simulink model "Combined_Power_Circuit"  (R2022b)
settings: Solver=VariableStepAuto  StartTime=0.0  StopTime=5  MaxStep=1e-5  RelTol=1e-3
libraries: spsDiodeLib x7, spsACVoltageSourceLib x3, spsCurrentMeasurementLib x3, spsVoltageMeasurementLib x2, spsDCMachineLib x1, spsMeanLib x1, spsMosfetLib x1, spspowerguiLib x1
settings Model: Creator=pc  LastModifiedBy=user
settings SolverCC: ZeroCrossAlgorithm=Adaptive
settings DebuggingCC: IgnoredZcDiagnostic=none  UnconnectedInputMsg=warning  UnconnectedOutputMsg=warning  UnconnectedLineMsg=warning
settings ModelReferenceCC: EnableRefExpFcnMdlSchedulingChecks=on
settings RTWCC: DLArmComputeVersion=19.05

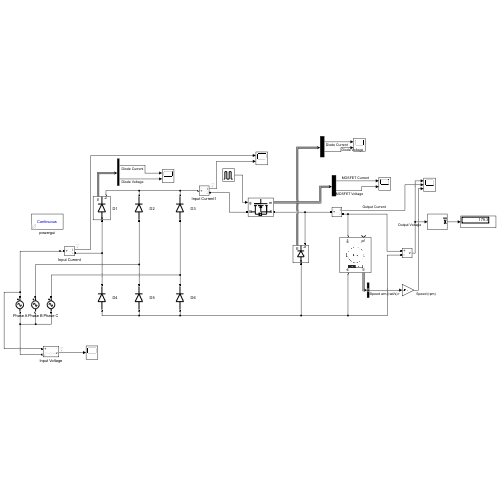
[thumbnail: Simulink's stored preview of the top-level diagram]
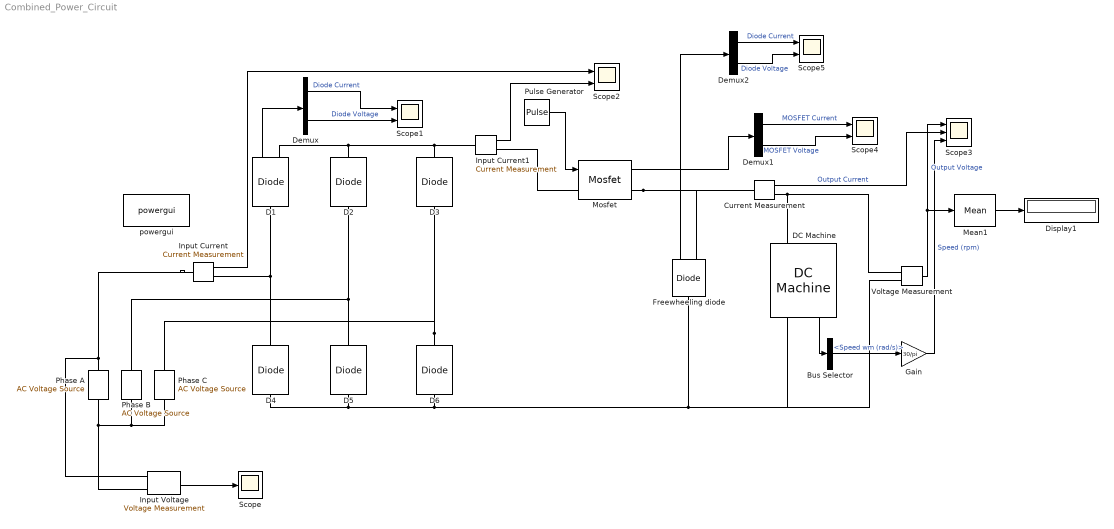
== system Combined_Power_Circuit ==
  " Phase A" : spsACVoltageSourceLib/AC Voltage Source  Amplitude=96.2*sqrt(2)  Phase=0  Frequency=50  SampleTime=0  Measurements=None  BusType=swing  Pref=10e3  Qref=0  Qmin=-inf  Qmax=+inf
  Bus Selector : BusSelector  OutputSignals=Speed wm (rad/s)
  Current Measurement : spsCurrentMeasurementLib/Current Measurement  PhasorSimulation=off  OutputType=Complex  PSBequivalent=0
  D1 : spsDiodeLib/Diode  Ron=0  Lon=0  Vf=0  IC=0  UseSnubber=0  Rs=inf  Cs=0  Measurements=on
  D{2..6} (5 alike) : spsDiodeLib/Diode  Ron=0  Lon=0  Vf=0  IC=0  UseSnubber=0  Rs=inf  Cs=0  Measurements=off
  DC Machine : spsDCMachineLib/DC Machine  PresetModel=No  MechanicalLoad=Torque TL  FieldType=Permanent magnet  ShowDetailedParameters=on  MeasurementBus=off  RLa="[ 0.8  0.0125]"  RLf="[ 210  23]"  Laf=1.8  MachineConstant=Back-emf constant (V/rpm)  Ke=220/1500  Kt=1.8  J=1  Bm=0  Tf=1.59  w0=0  Ifinit=1  TsPowergui=0  TsBlock=-1
  Demux : Demux  Outputs=2
  Demux1 : Demux  Outputs=2
  Demux2 : Demux  Outputs=2
  Display1 : Display
  Freewheeling diode : spsDiodeLib/Diode  Ron=0  Lon=0  Vf=0  IC=0  UseSnubber=off  Rs=inf  Cs=0  Measurements=on
  Gain : Gain  Gain=30/pi
  Input Current : spsCurrentMeasurementLib/Current Measurement  PhasorSimulation=off  OutputType=Complex  PSBequivalent=0
  Input Current1 : spsCurrentMeasurementLib/Current Measurement  PhasorSimulation=off  OutputType=Complex  PSBequivalent=0
  Input Voltage : spsVoltageMeasurementLib/Voltage Measurement  PhasorSimulation=off  OutputType=Complex  PSBequivalent=0
  Mean1 : spsMeanLib/Mean  Freq=60  Vinit=0  Ts=0
  Mosfet : spsMosfetLib/Mosfet  Ron=0.1  Lon=0  Rd=0.01  Vfd=0  IC=0  Rs=1e5  Cs=inf  Measurements=on
  Phase B : spsACVoltageSourceLib/AC Voltage Source  Amplitude=96.2*sqrt(2)  Phase=-120  Frequency=50  SampleTime=0  Measurements=None  BusType=swing  Pref=10e3  Qref=0  Qmin=-inf  Qmax=+inf
  Phase C : spsACVoltageSourceLib/AC Voltage Source  Amplitude=96.2*sqrt(2)  Phase=120  Frequency=50  SampleTime=0  Measurements=None  BusType=swing  Pref=10e3  Qref=0  Qmin=-inf  Qmax=+inf
  Pulse Generator : DiscretePulseGenerator  PulseType=Time based  Period=1/10000  PulseWidth=80
  Scope : Scope
  Scope{1..2,4..5} (4 alike) : Scope  NumInputPorts=2
  Scope3 : Scope  NumInputPorts=3
  Voltage Measurement : spsVoltageMeasurementLib/Voltage Measurement  PhasorSimulation=off  OutputType=Complex  PSBequivalent=0
  powergui : spspowerguiLib/powergui  Priority=1  SimulationMode=Continuous  SampleTime=50e-6  frequency=60  Iterations=50  frequencyindice=50  Pbase=100e6  ErrMax=1e-4  UnitsV=kV  UnitsW=MW  buscounter=0  FunctionMessages=off  echomessages=off  EnableUseOfTLC=off  CurrentSourceSwitches=off  DisableSnubberDevices=off  DisableRonSwitches=off  DisableVfSwitches=off  DisplayEquations=off  AutomaticDiscreteSolvers=off  SolverType=Tustin/Backward Euler (TBE)  Interpol=off  ExternalGateDelay=off  methode=off  Ts=100  x0status=blocks  SPID=on  SwTol=0  HookPort=off  NonlinearTolerance=1e-4  nMaxIteration=100  ContinueOnMaxIteration=off  RestoreLinks=warning  ResistiveCurrentMeasurement=off  Frange=[0:2:500]  Ylog=off  Xlog=on  ShowGrid=off  save=off  variable=ZData  structure=0  ZoomFFT=off  StartTime=0.0  cycles=1  DisplayStyle=1  fundamental=60  FreqAxis=off  MaxFrequency=1000  frequencyindicesteady=1  RmsSteady=1  display=off
  wires:
  Input Voltage/1 -> Scope/1
  D1/1 -> Demux/1
  Demux/1 -> Scope1/1  "Diode Current"
  Demux/2 -> Scope1/2  "Diode Voltage"
  Input Current1/1 -> Scope2/2
  Input Current/1 -> Scope2/1
  Current Measurement/1 -> Scope3/2  "Output Current"
  Pulse Generator/1 -> Mosfet/1
  Demux1/2 -> Scope4/2  "MOSFET Voltage"
  Freewheeling diode/1 -> Demux2/1
  Demux1/1 -> Scope4/1  "MOSFET Current"
  Demux2/2 -> Scope5/2  "Diode Voltage"
  Demux2/1 -> Scope5/1  "Diode Current"
  Mosfet/1 -> Demux1/1
  Voltage Measurement/1 -> Scope3/1, Mean1/1  "Output Voltage"
  Mean1/1 -> Display1/1
  DC Machine/1 -> Bus Selector/1
  Bus Selector/1 -> Gain/1  "<Speed wm (rad/s)>"
  Gain/1 -> Scope3/3  "Speed (rpm)"
  connections:
  D2/RConn1 -- Input Current1/LConn1 -- D3/RConn1 -- D1/RConn1
  D6/RConn1 -- D3/LConn1 -- Phase C/RConn1
  Input Current/RConn1 -- D1/LConn1 -- D4/RConn1
  D5/RConn1 -- D2/LConn1 -- Phase B/RConn1
  " Phase A"/RConn1 -- Input Current/LConn1 -- Input Voltage/LConn1
  " Phase A"/LConn1 -- Phase C/LConn1 -- Phase B/LConn1 -- Input Voltage/LConn2
  Mosfet/RConn1 -- Current Measurement/LConn1 -- Freewheeling diode/RConn1
  Voltage Measurement/LConn1 -- DC Machine/LConn1 -- Current Measurement/RConn1
  D6/LConn1 -- Voltage Measurement/LConn2 -- DC Machine/RConn1 -- Freewheeling diode/LConn1 -- D4/LConn1 -- D5/LConn1
  Input Current1/RConn1 -- Mosfet/LConn1
